simulink model "model_ex2"  (R2025b)
settings: Solver=VariableStepAuto  StartTime=0.0  StopTime=10.0  RelTol=1e-3
undefined symbols (not defined in the file): d, F, k, m
settings Model: Creator=mammadoo  LastModifiedBy=mammadoo

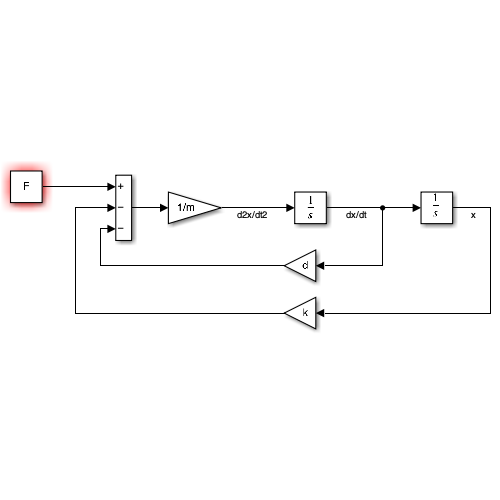
[thumbnail: Simulink's stored preview of the top-level diagram]
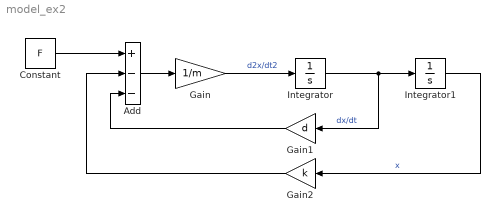
== system model_ex2 ==
  Add : Sum  Inputs=+--
  Constant : Constant  Value=F
  Gain : Gain  Gain=1/m
  Gain1 : Gain  Gain=d
  Gain2 : Gain  Gain=k
  Integrator : Integrator
  Integrator1 : Integrator
  wires:
  Add/1 -> Gain/1
  Integrator/1 -> Gain1/1, Integrator1/1  "dx/dt"
  Integrator1/1 -> Gain2/1  "x"
  Gain/1 -> Integrator/1  "d2x/dt2"
  Constant/1 -> Add/1
  Gain1/1 -> Add/3
  Gain2/1 -> Add/2
